simulink model "Cumulative_Sum_Ex2"  (R2025a)
settings: Solver=VariableStepAuto  StartTime=0.0  StopTime=511  RelTol=1e-3
undefined symbols (not defined in the file): S, vsva2197, xcvc1902
libraries: dspmathops x1, aieDSP x1, aieUtilities x1, vmcUtilities x1
settings Model: Creator=sdegala  LastModifiedBy=robg

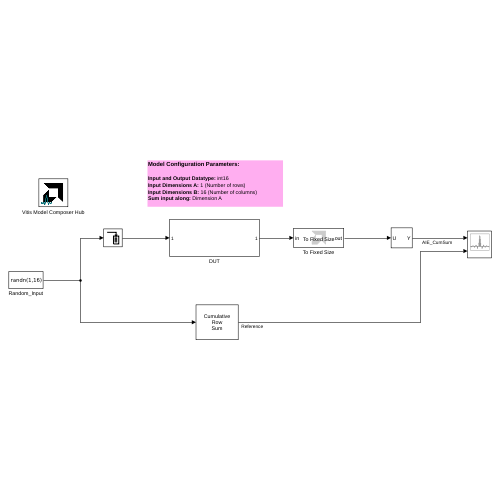
[thumbnail: Simulink's stored preview of the top-level diagram]
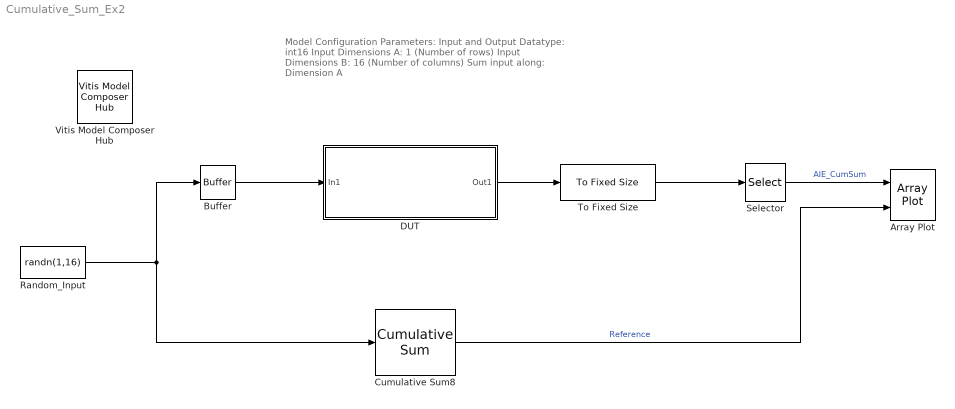
== system Cumulative_Sum_Ex2 ==
  note: Model Configuration Parameters:
      |
      | Input and Output Datatype: int16
      | Input Dimensions A: 1 (Number of rows)
      | Input Dimensions B: 16 (Number of columns)
      | Sum input along: Dimension A
  Array Plot : ArrayPlot  NumInputPorts=2  WindowPosition=[560.000000,350.000000,800.000000,500.000000,]  Visible=on  ScopeFrameLocation=window  YLimits=[-0.375 13.375]  ShowLegend=on
  Buffer : Buffer  N=256  OutputFrames=off
  Cumulative Sum8 : dspmathops/Cumulative Sum  dim=Rows  reset_popup=None  roundingMode=Floor  overflowMode=off  outputDataTypeStr=Inherit: Same as accumulator  outputMin=[]  outputMax=[]  outputLastDataTypeStr=Inherit: Same as accumulator
  DUT : Subsystem
  Random_Input : Constant  Value=randn(1,16)  OutDataTypeStr=int16  SampleTime=1
  Selector : Selector  InputPortWidth=256  IndexOptions=Index vector (dialog)  Indices=[1:1:16]  OutputSizes=1
  To Fixed Size : aieUtilities/To Fixed Size  Mode=Stop simulation when input variable-size signal is not full  OutputSize=Inherit: Same as input  CopyMethod=Buffer samples to form output  HasStatusOutput=on
  Vitis Model Composer Hub : vmcUtilities/Vitis Model Composer Hub  Tag=genX  CodeGeneration=off  StartColumn=1  NumberOfColumns=1  TargetDirectory=./code  exportDesign=off  analyzeDesign=off  validateDesignOnHw=off  ExportType=AI Engines  IpVendor=xilinx.com  IpLibrary=hls  IpVersion=1.0  IpHWLanguage=Verilog  AieCompilerOptions={}  AieSimulatorOptions={}  CreateTestbench=off  TestbenchStackSize=10  RunRtlSim=off  RunCSim=off  RunAieSim=off  enableSimulationTimeout=on  enableGraphIterations=on  AieSimTimeout=50000  AieGraphIterations=-1  RunAieSimProfiling=off  LaunchVitisAnalyzer=off  PlotOutput=off  RunX86Sim=off  X86SimTimeout=10  GenHwImage=off  GenLibadfXo=off  GenHwValidationCode=off  PlatformType=Specify Platform  Platform=/proj/xbuilds/SWIP/9999.0_0824_2321/installs/lin64/2025.2/Vitis/base_platforms/xilinx_vck190_base_202520_1/xilinx_vck190_base_202520_1.xpfm  HwSystemType=Baremetal  HwValidationTarget=hw  ProjDevice=Versal VCK190 Evaluation Platform (xcvc1902-vsva2197-2MP-e-S)  ProjDevicePart=xcvc1902-vsva2197-2MP-e-S  AIEType=AIE  SamplePeriod=-1  ClockFrequency=200  DataPathParallelism=1  xilinxfamily=versalaicore  part=xcvc1902  speed=-2MP-e-S  package=vsva2197  directory=./netlist  testbench=off  incr_netlist=off  synthesis_tool=Vivado  clock_wrapper=Clock Enables  dbl_ovrd=According to Block Masks  dcm_input_clock_period=10  sysclk_period=10  simulink_period=1  eval_field=0  LogFileName=''  NThreads=4
  wires:
  DUT/1(Out1) -> To Fixed Size/1
  To Fixed Size/1 -> Selector/1
  Random_Input/1 -> Buffer/1, Cumulative Sum8/1
  Buffer/1 -> DUT/1(In1)
  Selector/1 -> Array Plot/1  "AIE_CumSum"
  Cumulative Sum8/1 -> Array Plot/2  "Reference"

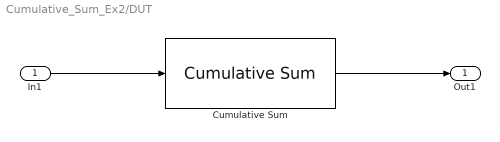
== system Cumulative_Sum_Ex2/DUT ==
  In1 : Inport
  Cumulative Sum : aieDSP/Cumulative Sum  AIE_VARIANT=1  data_type_in=int16  data_type_out=int16  dim_a=1  dim_b=16  num_frames=1  sum_mode=Dimension A  shift_output=0  rnd_mode=Floor  sat_mode=None  blockJsonConstraints=[]  blockJsonConstraintsInternal=[]  spec=vmc_cumsum.json  SerializedMaskParamNames=[]  SerializedMaskParamValues=[]  SerializedMaskParamVisibilities=[]  block_type=Cumulative Sum  SerializedMaskParamDataypes=uint|typename|typename|uint|uint|uint|uint|uint|uint|uint  SerializedMaskParamEnumStrArr=0|0|0|0|0|0|Dimension A,Dimension B|0|Floor,Ceiling,Round to positive infinity,Round to negative infinity,Round symmetrical to infinity,Round symmetrical to zero,Round convergent to even,Round convergent to odd|None,Saturate,Symmetric  SerializedMaskParamEnumValArr=0|0|0|0|0|0|0,1|0|0,1,2,3,4,5,6,7|0,1,3  SerializedMaskParamVectorArr=0|0|0|0|0|0|0|0|0|0  SerializedMaskParamKeys=AIE_VARIANT|TT_DATA|TT_OUT_DATA|TP_DIM_A|TP_DIM_B|TP_NUM_FRAMES|TP_MODE|TP_SHIFT|TP_RND|TP_SAT
  Out1 : Outport
  wires:
  In1/1 -> Cumulative Sum/1
  Cumulative Sum/1 -> Out1/1
